simulink model "aerodynamic_model"  (R2021a)
settings: configuration reference "Configuration" (kept outside this file)
undefined symbols (not defined in the file): C_D, rho
settings Model: DataDictionary=shared_config.sldd  Creator=francois  LastModifiedBy=esl
settings ConfigSetRef: SourceName=Configuration

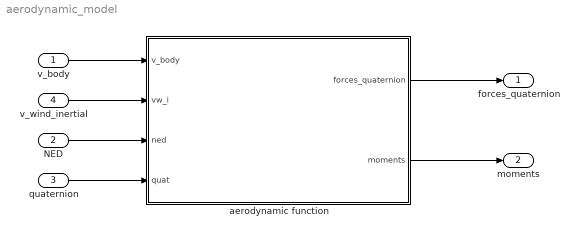
== system aerodynamic_model ==
  v_body : Inport  PortDimensions=3
  NED : Inport  Port=2  PortDimensions=3
  quaternion : Inport  Port=3  PortDimensions=4
  v_wind_inertial : Inport  Port=4  PortDimensions=3
  "aerodynamic function " : MATLAB Function  TreatAsAtomicUnit=on
  forces_quaternion : Outport
  "moments " : Outport  Port=2
  wires:
  "aerodynamic function "/2(moments) -> "moments "/1
  "aerodynamic function "/1(forces_quaternion) -> forces_quaternion/1
  v_body/1 -> "aerodynamic function "/1(v_body)
  v_wind_inertial/1 -> "aerodynamic function "/2(vw_i)
  NED/1 -> "aerodynamic function "/3(ned)
  quaternion/1 -> "aerodynamic function "/4(quat)

== matlab function aerodynamic_model/aerodynamic function  ==
  data: v_body input; forces_quaternion output; vw_i input; ned input; quat input; moments output; rho parameter size=1; C_D parameter size=3
function [forces_quaternion, moments] = aerodynamicModel(v_body, vw_i, ned, quat, rho, C_D)
    coder.extrinsic("quatrotate");
    
    % Initialize
    vw_b_quat = [0; 0; 0];
    
    vw_b_quat = quatrotate(quat', vw_i')';
    
    v_wb_relative_quat = -v_body + vw_b_quat;
    
    %q = 0.5 * rho * abs(v_bw).*v_bw;
    
    forces_quaternion = (0.5 * rho * abs(v_wb_relative_quat).*v_wb_relative_quat).*C_D;

    moments = [0; 0; 0];
    
end
